simulink subsystem "DM_ETBModel"  (R2019b)
settings: Solver=VariableStepAuto  StartTime=0.0  StopTime=10.0  RelTol=1e-3
undefined symbols (not defined in the file): DiscIntNeverNeededParam, model_springConstant, model_springPreload
libraries: simulink x1
settings Model: Creator=Nick  LastModifiedBy=Nick

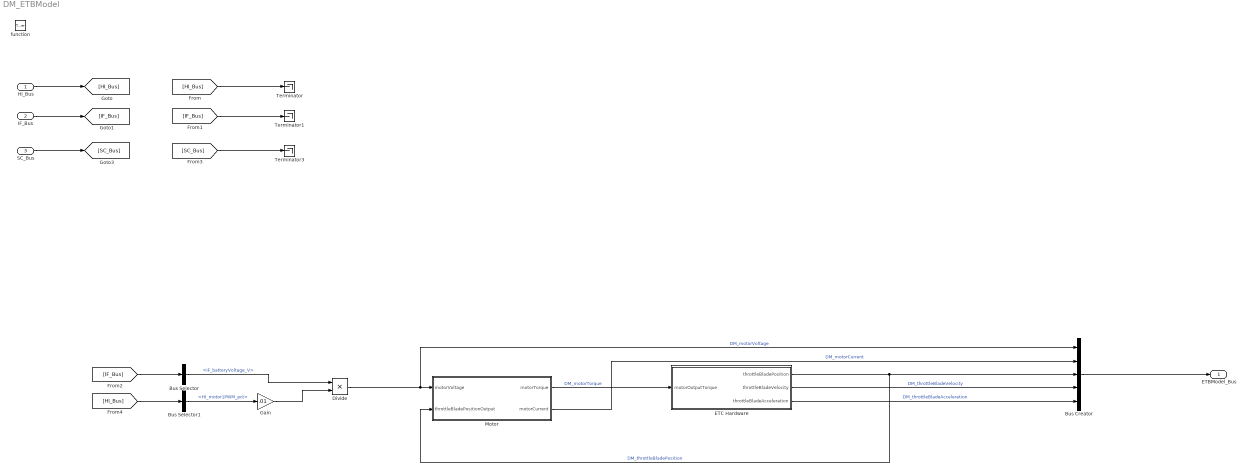
== system DM_ETBModel ==
  HI_Bus : Inport
  IF_Bus : Inport  Port=2
  SC_Bus : Inport  Port=3
  function : TriggerPort  TriggerType=function-call  VariantControl=Variant
  Bus Creator : BusCreator  Inputs=5
  Bus Selector : BusSelector  OutputSignals=AnalogInputFiltering_Bus.OnboardADCBus.IF_batteryVoltage_V
  Bus Selector1 : BusSelector  OutputSignals=VectorBoxBus.HI_motor1PWM_pct
  Divide : Product  Inputs=**
  ETC Hardware : Subsystem
  Gain : Gain  Gain=.01
  Motor : Subsystem
  Terminator : Terminator
  Terminator1 : Terminator
  Terminator3 : Terminator
  ETBModel_Bus : Outport
  wires:
  Gain/1 -> Divide/2
  Bus Selector1/1 -> Gain/1  "<HI_motor1PWM_pct>"
  [HI_Bus] -> Bus Selector1/1
  Bus Selector/1 -> Divide/1  "<IF_batteryVoltage_V>"
  ETC Hardware/3(throttleBladeAcceleration) -> Bus Creator/5  "DM_throttleBladeAcceleration"
  ETC Hardware/2(throttleBladeVelocity) -> Bus Creator/4  "DM_throttleBladeVelocity"
  ETC Hardware/1(throttleBladePosition) -> Bus Creator/3, Motor/2(throttleBladePositionOutput)  "DM_throttleBladePosition"
  Motor/1(motorTorque) -> ETC Hardware/1(motorOutputTorque)  "DM_motorTorque"
  Motor/2(motorCurrent) -> Bus Creator/2  "DM_motorCurrent"
  Divide/1 -> Motor/1(motorVoltage), Bus Creator/1  "DM_motorVoltage"
  [IF_Bus] -> Terminator1/1
  [HI_Bus] -> Terminator/1
  IF_Bus/1 -> [IF_Bus]
  HI_Bus/1 -> [HI_Bus]
  [SC_Bus] -> Terminator3/1
  SC_Bus/1 -> [SC_Bus]
  Bus Creator/1 -> ETBModel_Bus/1
  [IF_Bus] -> Bus Selector/1

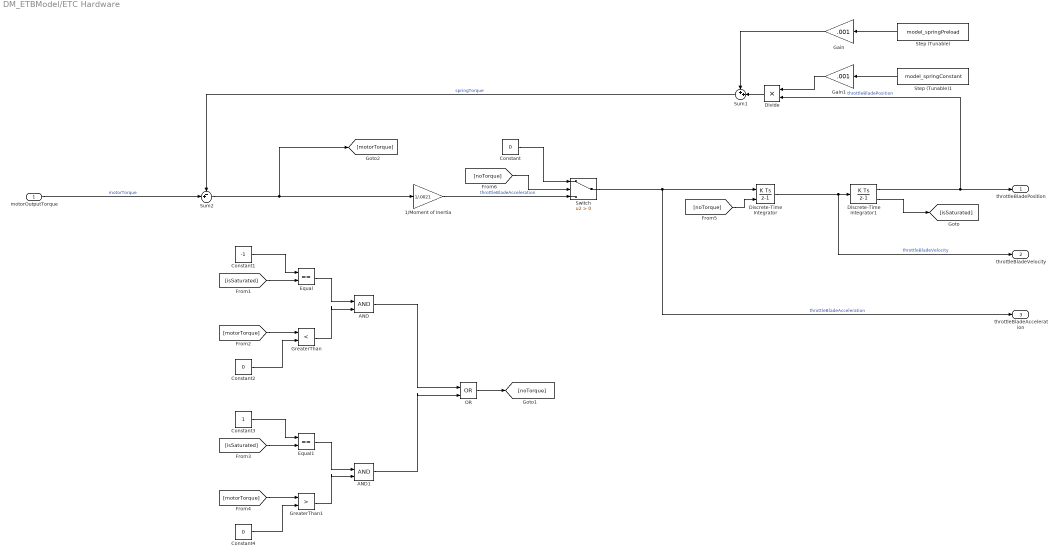
== system DM_ETBModel/ETC Hardware ==
  motorOutputTorque : Inport
  1/Moment of Inertia : Gain  Gain=1/.0021
  AND : Logic  IconShape=distinctive  AllPortsSameDT=off  OutDataTypeStr=boolean
  AND1 : Logic  IconShape=distinctive  AllPortsSameDT=off  OutDataTypeStr=boolean
  Constant : Constant  Value=0
  Constant1 : Constant  Value=-1
  Constant2 : Constant  Value=0
  Constant3 : Constant
  Constant4 : Constant  Value=0
  Discrete-Time Integrator : DiscreteIntegrator  ExternalReset=level  SampleTime=-1  ICPrevOutput=DiscIntNeverNeededParam  ICPrevScaledInput=DiscIntNeverNeededParam
  Discrete-Time Integrator1 : DiscreteIntegrator  SampleTime=-1  LimitOutput=on  UpperSaturationLimit=1.5708  LowerSaturationLimit=0  ShowSaturationPort=on  ICPrevOutput=DiscIntNeverNeededParam  ICPrevScaledInput=DiscIntNeverNeededParam
  Divide : Product  Inputs=**
  Equal : RelationalOperator  Operator===  OutDataTypeStr=boolean  RndMeth=Simplest
  Equal1 : RelationalOperator  Operator===  OutDataTypeStr=boolean  RndMeth=Simplest
  Gain : Gain  Gain=.001
  Gain1 : Gain  Gain=.001
  GreaterThan : RelationalOperator  Operator=<  OutDataTypeStr=boolean  RndMeth=Simplest
  GreaterThan1 : RelationalOperator  Operator=>  OutDataTypeStr=boolean  RndMeth=Simplest
  OR : Logic  Operator=OR  IconShape=distinctive  AllPortsSameDT=off  OutDataTypeStr=boolean
  Step (Tunable) : Constant  Value=model_springPreload  VectorParams1D=off  SampleTime=-1
  Step (Tunable)1 : Constant  Value=model_springConstant  VectorParams1D=off  SampleTime=-1
  Sum1 : Sum  Inputs=++|
  Sum2 : Sum  Inputs=-+|
  Switch : Switch  Criteria=u2 > Threshold
  throttleBladePosition : Outport
  throttleBladeVelocity : Outport  Port=2
  throttleBladeAcceleration : Outport  Port=3
  wires:
  Constant/1 -> Switch/1
  [noTorque] -> Switch/2
  1/Moment of Inertia/1 -> Switch/3  "throttleBladeAcceleration"
  [noTorque] -> Discrete-Time Integrator/2
  AND1/1 -> OR/2
  AND/1 -> OR/1
  GreaterThan1/1 -> AND1/2
  Equal1/1 -> AND1/1
  Constant3/1 -> Equal1/1
  [isSaturated] -> Equal1/2
  Constant4/1 -> GreaterThan1/2
  [motorTorque] -> GreaterThan1/1
  [motorTorque] -> GreaterThan/1
  Constant2/1 -> GreaterThan/2
  GreaterThan/1 -> AND/2
  [isSaturated] -> Equal/2
  OR/1 -> [noTorque]
  Discrete-Time Integrator1/2 -> [isSaturated]
  Equal/1 -> AND/1
  Constant1/1 -> Equal/1
  Sum2/1 -> [motorTorque], 1/Moment of Inertia/1
  Gain/1 -> Sum1/1
  Divide/1 -> Sum1/2
  Discrete-Time Integrator1/1 -> Divide/2, throttleBladePosition/1  "throttleBladePosition"
  Discrete-Time Integrator/1 -> Discrete-Time Integrator1/1, throttleBladeVelocity/1  "throttleBladeVelocity"
  Switch/1 -> throttleBladeAcceleration/1, Discrete-Time Integrator/1  "throttleBladeAcceleration"
  Sum1/1 -> Sum2/1  "springTorque"
  motorOutputTorque/1 -> Sum2/2  "motorTorque"
  Step (Tunable)/1 -> Gain/1
  Gain1/1 -> Divide/1
  Step (Tunable)1/1 -> Gain1/1

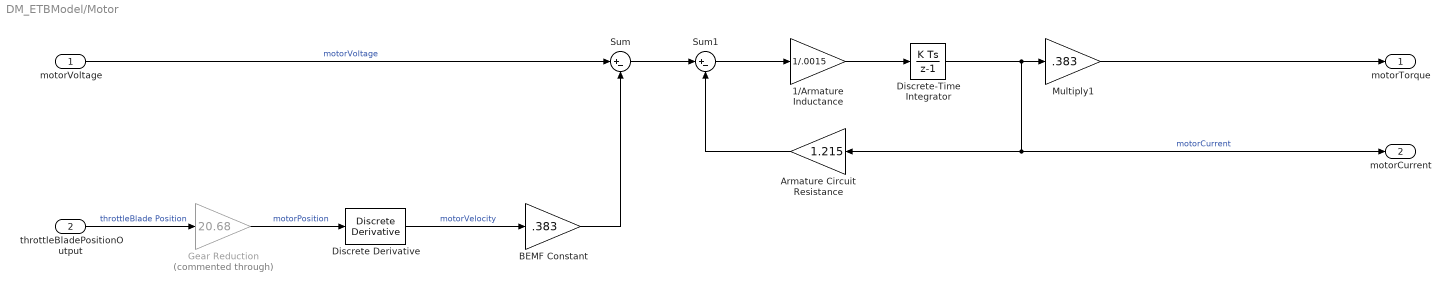
== system DM_ETBModel/Motor ==
  motorVoltage : Inport
  throttleBladePositionOutput : Inport  Port=2
  1/Armature Inductance : Gain  Gain=1/.0015
  Armature Circuit Resistance : Gain  Gain=1.215
  BEMF Constant : Gain  Gain=.383
  Discrete Derivative : simulink/Discrete/Discrete Derivative  gainval=1.0  ICPrevScaledInput=0.0  OutMin=[]  OutMax=[]  OutDataType=fixdt(1, 16)  OutScaling=2^-10  DoSatur=off
  Discrete-Time Integrator : DiscreteIntegrator  SampleTime=-1  ICPrevOutput=DiscIntNeverNeededParam  ICPrevScaledInput=DiscIntNeverNeededParam
  Gear Reduction : Gain  Commented=through  Gain=20.68
  Multiply1 : Gain  Gain=.383
  Sum : Sum  Inputs=|+-
  Sum1 : Sum  Inputs=|+-
  motorTorque : Outport
  motorCurrent : Outport  Port=2
  wires:
  Discrete Derivative/1 -> BEMF Constant/1  "motorVelocity"
  Gear Reduction/1 -> Discrete Derivative/1  "motorPosition"
  throttleBladePositionOutput/1 -> Gear Reduction/1  "throttleBlade Position"
  BEMF Constant/1 -> Sum/2
  Sum/1 -> Sum1/1
  1/Armature Inductance/1 -> Discrete-Time Integrator/1
  Sum1/1 -> 1/Armature Inductance/1
  Armature Circuit Resistance/1 -> Sum1/2
  motorVoltage/1 -> Sum/1  "motorVoltage"
  Multiply1/1 -> motorTorque/1
  Discrete-Time Integrator/1 -> Multiply1/1, motorCurrent/1, Armature Circuit Resistance/1  "motorCurrent"
